simulink model "ques_2_1_notch_simulink"  (R2023b)
settings: Solver=ode1  StartTime=0.0  StopTime=30.0  FixedStep=0.001  RelTol=1e-3
values from neighbouring files (symbols this model uses):
  beta1 = 0.01*10    (= 0.1)    [ques_2_1_notch.m]
  beta2 = 1    [ques_2_1_notch.m]
  f1 = 40    [ques_2_1_notch.m]
  f2 = 40    [ques_2_1_notch.m]
libraries: simulink x1
settings Model: Creator=sarth  LastModifiedBy=sarth

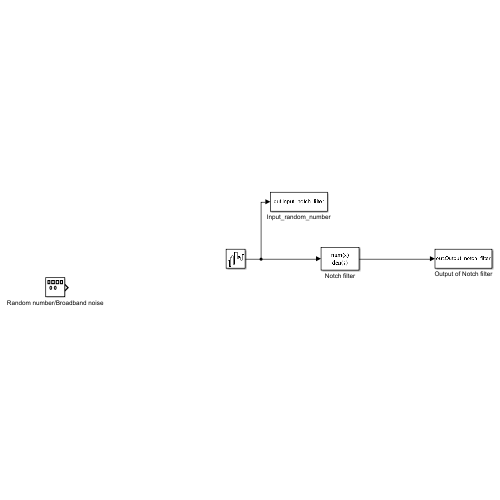
[thumbnail: Simulink's stored preview of the top-level diagram]
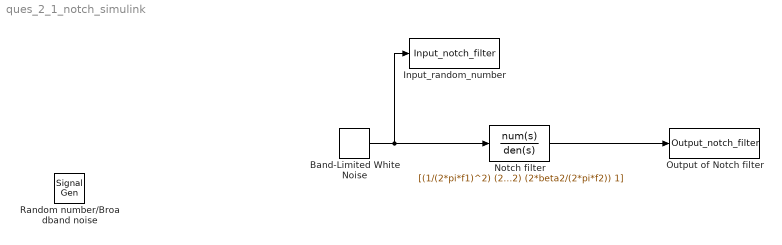
== system ques_2_1_notch_simulink ==
  Band-Limited White Noise : simulink/Sources/Band-Limited White Noise  Cov=[0.1]  Ts=0.001  seed=[23341]
  Input_random_number : ToWorkspace  VariableName=Input_notch_filter  SaveFormat=Timeseries  SampleTime=-1
  Notch filter : TransferFcn  Numerator=[(1/(2*pi*f1)^2) (2*beta1/(2*pi*f1)) 1 ]  Denominator=[(1/(2*pi*f2)^2) (2*beta2/(2*pi*f2)) 1]
  Output of Notch filter : ToWorkspace  VariableName=Output_notch_filter  SaveFormat=Timeseries  SampleTime=-1
  Random number/Broadband noise : SignalGenerator  WaveForm=random  Units=rad/sec
  wires:
  Band-Limited White Noise/1 -> Notch filter/1, Input_random_number/1
  Notch filter/1 -> Output of Notch filter/1
